simulink model "ES101A_DiagcMgr"  (R2013b)
settings: Solver=ode45  StartTime=0.0  StopTime=0.44  RelTol=1e-3
values from neighbouring files (symbols this model uses):
  BrdgVltg = DataDict.IpSignal    [ES101A_DiagcMgr_DataDict.m]
  DEM_CLEAR_PENDING = DataDict.Constant    [ES101A_DiagcMgr_DataDict.m]
  DEM_DTC_GROUP_ALL_DTCS = DataDict.Constant    [ES101A_DiagcMgr_DataDict.m]
  DFTAGICNTR_CNT_U08 = DataDict.Constant    [ES101A_DiagcMgr_DataDict.m]
  DIAGCMGR_NTCINFOSTSTESTFAILD_CNT_U08 = DataDict.Constant    [ES101A_DiagcMgr_DataDict.m]
  DIAGCMGR_NTCINFOSTSTESTFAILDTHISIGNCYC_CNT_U08 = DataDict.Constant    [ES101A_DiagcMgr_DataDict.m]
  DIAGCMGR_NTCINFOSTSTESTNOTCMPLTHISIGNCYC_CNT_U08 = DataDict.Constant    [ES101A_DiagcMgr_DataDict.m]
  DiagcMgrFltResp = DataDict.Calibration    [ES101A_DiagcMgr_DataDict.m]
  DiagcMgrNtcFltAry = DataDict.NVM    [ES101A_DiagcMgr_DataDict.m]
  DIAGCSTSCTRLDSHTDWNFLTPRSNT_CNT_U16 = DataDict.Constant    [ES101A_DiagcMgr_DataDict.m]
  DIAGCSTSDFTHWAG_CNT_U16 = DataDict.Constant    [ES101A_DiagcMgr_DataDict.m]
  DIAGCSTSDFTHWAGSERLCOMEXPRTVAL_CNT_U16 = DataDict.Constant    [ES101A_DiagcMgr_DataDict.m]
  DIAGCSTSDFTVEHSPD_CNT_U16 = DataDict.Constant    [ES101A_DiagcMgr_DataDict.m]
  DIAGCSTSININVAL_CNT_U16 = DataDict.Constant    [ES101A_DiagcMgr_DataDict.m]
  DIAGCSTSIVTR1INACTV_CNT_U16 = DataDict.Constant    [ES101A_DiagcMgr_DataDict.m]
  DIAGCSTSIVTR2INACTV_CNT_U16 = DataDict.Constant    [ES101A_DiagcMgr_DataDict.m]
  DIAGCSTSLIMDTPRFMNC_CNT_U16 = DataDict.Constant    [ES101A_DiagcMgr_DataDict.m]
  DIAGCSTSRAMPTOZEROFLTPRSNT_CNT_U16 = DataDict.Constant    [ES101A_DiagcMgr_DataDict.m]
  DIAGCSTSWHLIMBREJCTNDI_CNT_U16 = DataDict.Constant    [ES101A_DiagcMgr_DataDict.m]
  DTCIDXSTSFAIL_CNT_U08 = DataDict.Constant    [ES101A_DiagcMgr_DataDict.m]
  DTCIDXSTSNONTC_CNT_U08 = DataDict.Constant    [ES101A_DiagcMgr_DataDict.m]
  DTCIDXSTSNORES_CNT_U08 = DataDict.Constant    [ES101A_DiagcMgr_DataDict.m]
  DTCIDXSTSPASS_CNT_U08 = DataDict.Constant    [ES101A_DiagcMgr_DataDict.m]
  DTCIDXSTSUPDCFMD_CNT_U08 = DataDict.Constant    [ES101A_DiagcMgr_DataDict.m]
  ELECGLBPRM_IVTRCNT_CNT_U08 = DataDict.ConfigParam    [ES101A_DiagcMgr_DataDict.m]
  FLTINJ_DIAGCMGR_DIAGCSTSIVTR1INACTV = DataDict.Constant    [ES101A_DiagcMgr_DataDict.m]
  FLTINJ_DIAGCMGR_DIAGCSTSIVTR2INACTV = DataDict.Constant    [ES101A_DiagcMgr_DataDict.m]
  HwTq = DataDict.IpSignal    [ES101A_DiagcMgr_DataDict.m]
  IgnCntr = DataDict.IpSignal    [ES101A_DiagcMgr_DataDict.m]
  MAXDEBCNTRVAL_CNT_S16 = DataDict.Constant    [ES101A_DiagcMgr_DataDict.m]
  MAXRAMPRATE_ULSPERSEC_F32 = DataDict.Constant    [ES101A_DiagcMgr_DataDict.m]
  MINDEBCNTRVAL_CNT_S16 = DataDict.Constant    [ES101A_DiagcMgr_DataDict.m]
  MINRAMPRATE_ULSPERSEC_F32 = DataDict.Constant    [ES101A_DiagcMgr_DataDict.m]
  SCAMOTTQCMDTOONE_ULS_F32 = DataDict.Constant    [ES101A_DiagcMgr_DataDict.m]
  SCAMOTTQCMDTOZERO_ULS_F32 = DataDict.Constant    [ES101A_DiagcMgr_DataDict.m]
  SysSt = DataDict.IpSignal    [ES101A_DiagcMgr_DataDict.m]
  VehSpd = DataDict.IpSignal    [ES101A_DiagcMgr_DataDict.m]
undefined symbols (not defined in the file or in its folder): ActvMotTqCmdSca, ActvRampRate, AgiCntr, Dem_DTCFormatType, Dem_DTCOriginType, Dem_EventStatusType, DiagcData, DiagcMgrNtcMap, DiagcSts, DtcEnaMask, EcuT, HistNtcFltAry, MicroDiagcData, MotTq, NtcNr, NtcNrWithResd1, NtcStInfo, ProxySetNtcData, Sts, SysSt1, TOTNROFDTC_CNT_U08
libraries: simulink x151, FloatToFixd x5, NxtrNvM x4
(part 2 of 13)

== system ES101A_DiagcMgr/DiagcMgr/ClrSnpshtData ==
  Function : TriggerPort  TriggerType=function-call  OutputDataType=double
  Constant : Constant  OutDataTypeStr=uint8
  CopyRight2 : Subsystem  Description=|  mask(Copyright Information){none=on}
      | Copyright info block.                                               
      |                                                                     
      | Place copyright information at the top of every subsystem in design.
      mask prompts: none "No parameters"
      mask help: Place copyright information at the top of every subsystem in design.
      mask Display:
      | NxtrConf = 'Nexteer Confidential';
      | 
      | sys = bdroot; %handle for the current model ("system")
      | first = get_param(sys,'Created');
      | first = first(end-3:end);  %year is last four digits
      | 
      | last = get_param(sys,'LastModifiedDate');
      | if isempty(last)
      |     last = datestr(now,'yyyy');
      | else
      |     last = last(end-3:end);
      | end
      | 
      | if strcmp(first,last)
      |     fprintf('%s -- Copyright %s Nexteer',NxtrConf,first)
      | else
      |     fprintf('%s -- %s%s- %s Nexteer',NxtrConf,char(169),first,last)
      | end
  Data Store Read1 : DataStoreRead  DataStoreName=SnpshtDataAry
  Set Ram Block Status : NxtrNvM/Set Ram Block Status  FuncName=Set Ram Block Status  NvMBlockName=SnpShtDataAry  VoidFuncRtn=on  BlockChanged_DSN=NvMSRBS_BlockChanged  Return_DSN=NvMSRBS_Return
      settings: AttributesFormatString=%<FuncName>
  Subsystem : Subsystem
  Width : Width  DataType=uint8
  wires:
  Width/1 -> Subsystem/1(Length of Snapshot Array)
  Data Store Read1/1 -> Width/1
  Constant/1 -> Set Ram Block Status/1

== system ES101A_DiagcMgr/DiagcMgr/CopyRight2 ==

== system ES101A_DiagcMgr/DiagcMgr/DiagcMgrIninCore ==
  note: ProxySetNtcData and DiagcData
      | are not inputs, outputs or arguments to the
      | DiagcMgrIninCore. They are being used for
      | modelling purpose to show that the data is
      | being written to the respective structs.
  AppIdx_ArgIn : Inport
  NtcInfoArySize : Inport  Port=2
  NtcInfoAry_ArgIn : Inport  Port=3
  DiagcData : Inport  Port=4
  ProxySetNtcData : Inport  Port=5
  Function : TriggerPort  TriggerType=function-call  OutputDataType=double
  CopyRight2 : Subsystem  Description=|  mask(Copyright Information){none=on}
      | Copyright info block.                                               
      |                                                                     
      | Place copyright information at the top of every subsystem in design.
      mask prompts: none "No parameters"
      mask help: Place copyright information at the top of every subsystem in design.
      mask Display:
      | NxtrConf = 'Nexteer Confidential';
      | 
      | sys = bdroot; %handle for the current model ("system")
      | first = get_param(sys,'Created');
      | first = first(end-3:end);  %year is last four digits
      | 
      | last = get_param(sys,'LastModifiedDate');
      | if isempty(last)
      |     last = datestr(now,'yyyy');
      | else
      |     last = last(end-3:end);
      | end
      | 
      | if strcmp(first,last)
      |     fprintf('%s -- Copyright %s Nexteer',NxtrConf,first)
      | else
      |     fprintf('%s -- %s%s- %s Nexteer',NxtrConf,char(169),first,last)
      | end
  Initialize the NtcInfo Array : Subsystem  Priority=2
      settings: AttributesFormatString=Priority = %<Priority>
  Update DiagcSts and DiagcMgrActv : Subsystem  RequirementInfo="{'linktype_rmi_doors' '0000c474 (/ESG Group/FDD Module Requirements/EA4 Specific/ES101A_DiagcMgr)' '#ES101A_288' 'true' 'REQ:  ES101A_288' '' ; 'linktype_rmi_doors' '0000c474 (/ESG Group/FDD Module Requirements/EA4 Specific/ES101A_DiagcMgr)' '#ES101A_147' 'true' 'REQ:  ES101A_147' '' } %GIDa_8493db0a_cdf8_4c0c_9032_5c31bd2188ab"  Priority=3
      settings: AttributesFormatString=Priority = %<Priority>
  Update NtcInfoAry From NvM : Subsystem  Priority=1
      settings: AttributesFormatString=Priority = %<Priority>
  ProxySetNtcData_ArgOut : Outport
  DiagcData_ArgOut : Outport  Port=2
  NtcInfoAry_ArgOut : Outport  Port=3
  wires:
  Update DiagcSts and DiagcMgrActv/1(ProxySetNtcData_ArgOut) -> ProxySetNtcData_ArgOut/1
  Update DiagcSts and DiagcMgrActv/2(DiagcData_ArgOut) -> DiagcData_ArgOut/1
  NtcInfoArySize/1 -> Initialize the NtcInfo Array/1(NtcInfoArySize)
  Initialize the NtcInfo Array/1(NtcInfoAry_ArgOut) -> NtcInfoAry_ArgOut/1
  AppIdx_ArgIn/1 -> Update NtcInfoAry From NvM/1(AppIdx_ArgIn)
  NtcInfoAry_ArgIn/1 -> Update NtcInfoAry From NvM/2(NtcInfoAry_ArgIn)
  ProxySetNtcData/1 -> Update DiagcSts and DiagcMgrActv/1(ProxySetNtcData)
  DiagcData/1 -> Update DiagcSts and DiagcMgrActv/2(DiagcData)
  Update NtcInfoAry From NvM/1(NtcInfoAry_ArgOut) -> [NtcInfoAry]
  [NtcInfoAry] -> Initialize the NtcInfo Array/2(NtcInfoAry_ArgIn)

== system ES101A_DiagcMgr/DiagcMgr/DiagcMgrPer1 ==
  note: SysDiRampRate and SysDiMotTqCmdSca have their initial output set as
      | 0.1 UlsPerSec and 1 respectively.
  note: Design Consideration:
      |
      | ES101A_v2.X.0 assumes that no loop faster than 2ms can set faults.
      |
      | OutpDiagcSts, OutpActvRampRate and OutpActvMotTqCmdSca are initialized to
      | the default values.
      |
      | Default values of OutpDiagcSts is DIAGCSTSIVTR2INACTV_CNT_U16 if the program is a single inverter configuration.
      | else DIAGCSTSININVAL_CNT_U16 if the program is a dual inverter configuration.
      |
      | Default values of OutpRampRate is MINRAMPRATE_ULSPERSEC_F32.
      |
      | Default values of OutpMotTqCmdSca is SCAMOTTQCMDTOONE_ULS_F32.
      |
      | Need to call the server runnable GetDiagcDataApplX to get the DiagcMgrDiagcSts,
      | DiagcMgrActvRampRate and DiagcMgrActvMotTqCmdSca
      |
      | DiagcMgrPer1 udpates the OutpDiagcSts with the
      | ORed values of ALL application's DiagcMgrDiagcStsX
      |
      | DiagcMgrPer1 udpates the OutpActvRampRate with the
      | MAX value of ALL application's DiagcMgrRampRateX.
      |
      | DiagcMgrPer1 udpates the OutpActvMotTqCmdSca with the
      | MIN value of ALL application's DiagcMgrMotTqCmdScaX
  Function : TriggerPort  TriggerType=function-call
  CopyRight2 : Subsystem  Description=|  mask(Copyright Information){none=on}
      | Copyright info block.                                               
      |                                                                     
      | Place copyright information at the top of every subsystem in design.
      mask prompts: none "No parameters"
      mask help: Place copyright information at the top of every subsystem in design.
      mask Display:
      | NxtrConf = 'Nexteer Confidential';
      | 
      | sys = bdroot; %handle for the current model ("system")
      | first = get_param(sys,'Created');
      | first = first(end-3:end);  %year is last four digits
      | 
      | last = get_param(sys,'LastModifiedDate');
      | if isempty(last)
      |     last = datestr(now,'yyyy');
      | else
      |     last = last(end-3:end);
      | end
      | 
      | if strcmp(first,last)
      |     fprintf('%s -- Copyright %s Nexteer',NxtrConf,first)
      | else
      |     fprintf('%s -- %s%s- %s Nexteer',NxtrConf,char(169),first,last)
      | end
  Update OutpDiagcData : Subsystem  RequirementInfo={} %GIDa_85c462ac_a7f2_40f7_9507_c2fa4f4de765  Priority=2  TreatAsAtomicUnit=on
      settings: AttributesFormatString=|
      | Priority = %<Priority>
      | %<Description>
  Update the Reduced Performance Outputs : Subsystem  Priority=2
      settings: AttributesFormatString=Priority = %<Priority>
  SysDiRampRate : Outport  InitialOutput=0.1
  SysDiMotTqCmdSca : Outport  Port=2  OutMin=[0]  OutMax=[1]  InitialOutput=1
  SysStFltOutpReqDi : Outport  Port=3
  DiagcStsLimdTPrfmnc : Outport  Port=4
  DiagcStsIvtr1Inactv : Outport  Port=5
  DiagcStsIvtr2Inactv : Outport  Port=6
  DiagcStsDftHwAg : Outport  RequirementInfo={} %GIDa_cebdabc8_1fab_4827_8ce2_641fe406cf61  Port=7
  DiagcStsDftVehSpd : Outport  RequirementInfo={} %GIDa_5ce1feaf_f885_43d9_a11b_961b529a5fef  Port=8
  DiagcStsDftHwAgSerlComExprtVal : Outport  RequirementInfo={} %GIDa_e0e4e2a8_addf_43dd_a724_2e2318a08aac  Port=9
  DiagcStsWhlImbRejctnDi : Outport  RequirementInfo={} %GIDa_d2eab3b7_33f5_4627_ba04_dc7cade08e2d  Port=10
  DiagcStsCtrldShtDwnFltPrsnt : Outport  RequirementInfo={} %GIDa_78682114_6521_49d0_bf72_17a6b6e216ee  Port=11
  wires:
  Update the Reduced Performance Outputs/1(SysDiRampRate) -> SysDiRampRate/1
  Update the Reduced Performance Outputs/2(SysDiMotTqCmdSca) -> SysDiMotTqCmdSca/1
  Update the Reduced Performance Outputs/3(SysStFltOutpReqDi) -> SysStFltOutpReqDi/1
  Update the Reduced Performance Outputs/4(DiagcStsLimdTPrfmnc) -> DiagcStsLimdTPrfmnc/1
  Update the Reduced Performance Outputs/5(DiagcStsIvtr1Inactv) -> DiagcStsIvtr1Inactv/1
  Update the Reduced Performance Outputs/6(DiagcStsIvtr2Inactv) -> DiagcStsIvtr2Inactv/1
  Update the Reduced Performance Outputs/7(DiagcStsDftHwAg) -> DiagcStsDftHwAg/1
  Update the Reduced Performance Outputs/8(DiagcStsDftVehSpd) -> DiagcStsDftVehSpd/1
  Update the Reduced Performance Outputs/9(DiagcStsDftHwAgSerlComExprtVal) -> DiagcStsDftHwAgSerlComExprtVal/1
  Update the Reduced Performance Outputs/10(DiagcStsWhlImbRejctnDi) -> DiagcStsWhlImbRejctnDi/1
  Update the Reduced Performance Outputs/11(DiagcStsCtrldShtDwnFltPrsnt) -> DiagcStsCtrldShtDwnFltPrsnt/1
  Update OutpDiagcData/1(OutpDiagcSts) -> [OutpDiagcSts]
  Update OutpDiagcData/3(OutpMotTqCmdSca) -> [OutpMotTqCmdSca]
  Update OutpDiagcData/2(OutpRampRate) -> [OutpRampRate]
  [OutpRampRate] -> Update the Reduced Performance Outputs/2(OutpRampRate)
  [OutpMotTqCmdSca] -> Update the Reduced Performance Outputs/3(OutpMotTqCmdSca)
  [OutpDiagcSts] -> Update the Reduced Performance Outputs/1(OutpDiagcSts)

== system ES101A_DiagcMgr/DiagcMgr/DiagcMgrPer2 ==
  note: Limitation of the design:
      | Suppose, as an example, we have NTCs 5,6,7 and 8 mapped to a DTC 4:
      | If NTCs 5,6,7 have a status of NoRes and 8 Reaches a status of Failed, the DTC is
      | updated to show a status of Failed.
      | If the NTC 8 is a recoverable NTC, then happens to reach a state of Passed,
      | the DtcIdxSts will show a status of NoRes and the DEM will still show that the DTC has Failed.
  Function : TriggerPort  TriggerType=function-call
  Clear All DTCs : Subsystem  RequirementInfo="{'linktype_rmi_doors' '0000c474 (/ESG Group/FDD Module Requirements/EA4 Specific/ES101A_DiagcMgr)' '#ES101A_318' 'true' 'REQ:  ES101A_318' '' } %GIDa_daa6a456_375f_4596_a22c_ed37d4d53311"
  CopyRight2 : Subsystem  Description=|  mask(Copyright Information){none=on}
      | Copyright info block.                                               
      |                                                                     
      | Place copyright information at the top of every subsystem in design.
      mask prompts: none "No parameters"
      mask help: Place copyright information at the top of every subsystem in design.
      mask Display:
      | NxtrConf = 'Nexteer Confidential';
      | 
      | sys = bdroot; %handle for the current model ("system")
      | first = get_param(sys,'Created');
      | first = first(end-3:end);  %year is last four digits
      | 
      | last = get_param(sys,'LastModifiedDate');
      | if isempty(last)
      |     last = datestr(now,'yyyy');
      | else
      |     last = last(end-3:end);
      | end
      | 
      | if strcmp(first,last)
      |     fprintf('%s -- Copyright %s Nexteer',NxtrConf,first)
      | else
      |     fprintf('%s -- %s%s- %s Nexteer',NxtrConf,char(169),first,last)
      | end
  Data Store Read : DataStoreRead  DataStoreName=PrevClrDtcFlg
  Data Store Read1 : DataStoreRead  DataStoreName=ClrDiagcFlg
  If : If  NumInputs=2  IfExpression=u1 ~= u2
  Normal Periodic Processing : Subsystem  RequirementInfo="{'linktype_rmi_doors' '0000c474 (/ESG Group/FDD Module Requirements/EA4 Specific/ES101A_DiagcMgr)' '#ES101A_322' 'true' 'REQ:  ES101A_322' '' ; 'linktype_rmi_doors' '0000c474 (/ESG Group/FDD Module Requirements/EA4 Specific/ES101A_DiagcMgr)' '#ES101A_308' 'true' 'REQ:  ES101A_308' '' } %GIDa_fa1cf601_71d2_4de3_81ca_c465534cf8bb"
  wires:
  Data Store Read1/1 -> If/1
  Data Store Read/1 -> If/2
  If/1 -> Clear All DTCs/Action
  If/2 -> Normal Periodic Processing/Action

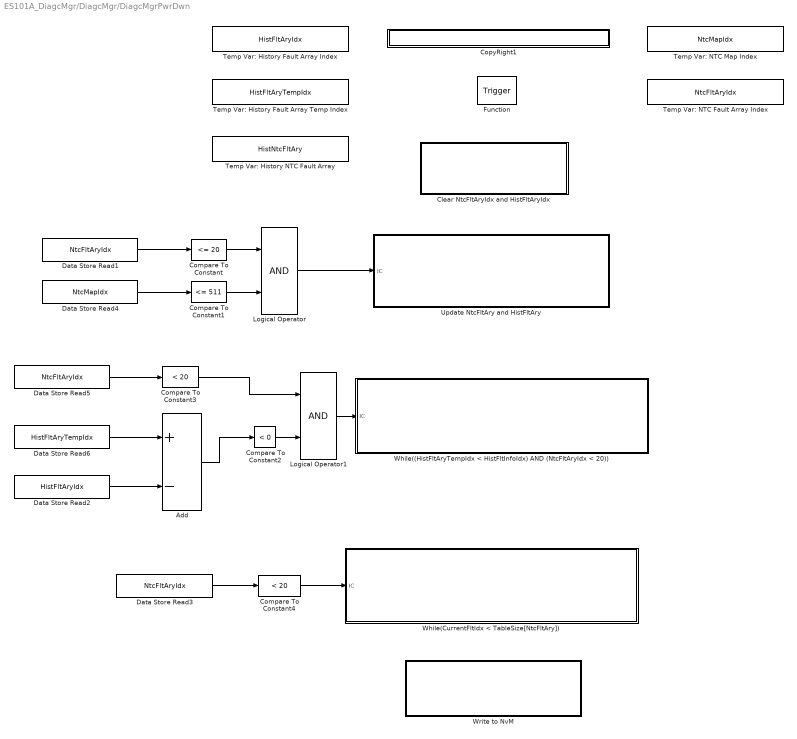
== system ES101A_DiagcMgr/DiagcMgr/DiagcMgrPwrDwn ==
  Function : TriggerPort  TriggerType=function-call
  Add : Sum  Inputs=+-
  Clear NtcFltAryIdx and HistFltAryIdx : Subsystem  Priority=1
      settings: AttributesFormatString=Priority = %<Priority>
  Compare To Constant : simulink/Logic and Bit Operations/Compare To Constant  relop=<=  const=20  OutDataTypeStr=boolean
  Compare To Constant1 : simulink/Logic and Bit Operations/Compare To Constant  relop=<=  const=511  OutDataTypeStr=boolean
  Compare To Constant2 : simulink/Logic and Bit Operations/Compare To Constant  relop=<  const=0  OutDataTypeStr=boolean
  Compare To Constant3 : simulink/Logic and Bit Operations/Compare To Constant  relop=<  const=20  OutDataTypeStr=boolean
  Compare To Constant4 : simulink/Logic and Bit Operations/Compare To Constant  relop=<  const=20  OutDataTypeStr=boolean
  CopyRight1 : Subsystem  Description=|  mask(Copyright Information){none=on}
      | Copyright info block.                                               
      |                                                                     
      | Place copyright information at the top of every subsystem in design.
      mask prompts: none "No parameters"
      mask help: Place copyright information at the top of every subsystem in design.
      mask Display:
      | NxtrConf = 'Nexteer Confidential';
      | 
      | sys = bdroot; %handle for the current model ("system")
      | first = get_param(sys,'Created');
      | first = first(end-3:end);  %year is last four digits
      | 
      | last = get_param(sys,'LastModifiedDate');
      | if isempty(last)
      |     last = datestr(now,'yyyy');
      | else
      |     last = last(end-3:end);
      | end
      | 
      | if strcmp(first,last)
      |     fprintf('%s -- Copyright %s Nexteer',NxtrConf,first)
      | else
      |     fprintf('%s -- %s%s- %s Nexteer',NxtrConf,char(169),first,last)
      | end
  Data Store Read1 : DataStoreRead  DataStoreName=NtcFltAryIdx
  Data Store Read2 : DataStoreRead  DataStoreName=HistFltAryIdx
  Data Store Read3 : DataStoreRead  DataStoreName=NtcFltAryIdx
  Data Store Read4 : DataStoreRead  DataStoreName=NtcMapIdx
  Data Store Read5 : DataStoreRead  DataStoreName=NtcFltAryIdx
  Data Store Read6 : DataStoreRead  DataStoreName=HistFltAryTempIdx
  Logical Operator : Logic  AllPortsSameDT=off  OutDataTypeStr=boolean
  Logical Operator1 : Logic  AllPortsSameDT=off  OutDataTypeStr=boolean
  Temp Var: History Fault Array Index : DataStoreMemory  DataStoreName=HistFltAryIdx  ReadBeforeWriteMsg=warning  WriteAfterWriteMsg=warning  WriteAfterReadMsg=warning  InitialValue=19  OutDataTypeStr=uint8
  Temp Var: History Fault Array Temp Index : DataStoreMemory  DataStoreName=HistFltAryTempIdx  ReadBeforeWriteMsg=warning  WriteAfterWriteMsg=warning  WriteAfterReadMsg=warning  InitialValue=1  OutDataTypeStr=uint8
  Temp Var: History NTC Fault Array : DataStoreMemory  RequirementInfo={} %GIDa_eaafd789_c2c3_4d7f_bafd_485e89611a26  DataStoreName=HistNtcFltAry  InitialValue=[0 0 0 0 0 0 0 0 0 0 0 0 0 0 0 0 0 0 0 0]  OutDataTypeStr=Bus: NtcFltInfoRec1  Dimensions=20
  Temp Var: NTC Fault Array Index : DataStoreMemory  DataStoreName=NtcFltAryIdx  ReadBeforeWriteMsg=warning  WriteAfterWriteMsg=warning  WriteAfterReadMsg=warning  InitialValue=19  OutDataTypeStr=uint8
  Temp Var: NTC Map Index : DataStoreMemory  DataStoreName=NtcMapIdx  ReadBeforeWriteMsg=warning  WriteAfterWriteMsg=warning  WriteAfterReadMsg=warning  InitialValue=1  OutDataTypeStr=uint8
  Update NtcFltAry and HistFltAry : Subsystem  Priority=2
      settings: AttributesFormatString=Priority = %<Priority>
  While((HistFltAryTempIdx < HistFltInfoIdx) AND (NtcFltAryIdx < 20)) : Subsystem  Priority=3  TreatAsAtomicUnit=on
      settings: AttributesFormatString=Priority = %<Priority>
  While(CurrentFltIdx < TableSize[NtcFltAry]) : Subsystem  Priority=4  TreatAsAtomicUnit=on
      settings: AttributesFormatString=Priority = %<Priority>
  Write to NvM : Subsystem  Priority=5
      settings: AttributesFormatString=Priority = %<Priority>
  wires:
  Data Store Read3/1 -> Compare To Constant4/1
  Compare To Constant4/1 -> While(CurrentFltIdx < TableSize[NtcFltAry])/1(IC)
  Logical Operator/1 -> Update NtcFltAry and HistFltAry/1(IC)
  Data Store Read1/1 -> Compare To Constant/1
  Compare To Constant/1 -> Logical Operator/1
  Compare To Constant1/1 -> Logical Operator/2
  Data Store Read4/1 -> Compare To Constant1/1
  Data Store Read6/1 -> Add/1
  Data Store Read2/1 -> Add/2
  Add/1 -> Compare To Constant2/1
  Data Store Read5/1 -> Compare To Constant3/1
  Compare To Constant3/1 -> Logical Operator1/1
  Logical Operator1/1 -> While((HistFltAryTempIdx < HistFltInfoIdx) AND (NtcFltAryIdx < 20))/1(IC)
  Compare To Constant2/1 -> Logical Operator1/2

== system ES101A_DiagcMgr/DiagcMgr/GetNtcActvCore  ==
  note: SW Implementation:
      |
      | 	SW uses a switched case with ApplIdx as the input. The GetNtcInfoApplX is
      | 	called inside each of the switched case statements. Based on the application
      | 	index, the respective NtcInfoAryX is selected.
  note: Design Rationale:
      |
      | 	If an NTC that is not configured in the NTC Map is called by any application/component,
      | 	its application index would be read as 255 and it enters the default case in the above switch
      | 	statement. This would indicate that the NTC has a Not Active State.
  NtcNr_ArgIn : Inport
  Function : TriggerPort  TriggerType=function-call
  Bus Selector : BusSelector  OutputSignals=Sts
  Bus Selector3 : BusSelector  OutputSignals=ApplIdx,NtcInfoIdx
  Compare to Zero : simulink/Logic and Bit Operations/Compare To Zero  relop=~=  OutDataTypeStr=boolean
  Compare to Zero1 : simulink/Logic and Bit Operations/Compare To Zero  relop=~=  OutDataTypeStr=boolean
  CopyRight2 : Subsystem  Description=|  mask(Copyright Information){none=on}
      | Copyright info block.                                               
      |                                                                     
      | Place copyright information at the top of every subsystem in design.
      mask prompts: none "No parameters"
      mask help: Place copyright information at the top of every subsystem in design.
      mask Display:
      | NxtrConf = 'Nexteer Confidential';
      | 
      | sys = bdroot; %handle for the current model ("system")
      | first = get_param(sys,'Created');
      | first = first(end-3:end);  %year is last four digits
      | 
      | last = get_param(sys,'LastModifiedDate');
      | if isempty(last)
      |     last = datestr(now,'yyyy');
      | else
      |     last = last(end-3:end);
      | end
      | 
      | if strcmp(first,last)
      |     fprintf('%s -- Copyright %s Nexteer',NxtrConf,first)
      | else
      |     fprintf('%s -- %s%s- %s Nexteer',NxtrConf,char(169),first,last)
      | end
  DIAGCMGR_NTCINFOSTSTESTFAILDTHISIGNCYC_CNT_U08 : simulink/Logic and Bit Operations/Bitwise Operator  logicop=AND  UseBitMask=on  BitMask=DIAGCMGR_NTCINFOSTSTESTFAILDTHISIGNCYC_CNT_U08  BitMaskRealWorld=Stored Integer
  DIAGCMGR_NTCINFOSTSTESTFAILD_CNT_U08 : simulink/Logic and Bit Operations/Bitwise Operator  logicop=AND  UseBitMask=on  BitMask=DIAGCMGR_NTCINFOSTSTESTFAILD_CNT_U08  BitMaskRealWorld=Stored Integer
  Data Store Read2 : DataStoreRead  DataStoreName=DiagcMgrNtcMap  DataStoreElements=DiagcMgrNtcMap(:)
  Data Type Conversion : DataTypeConversion  OutDataTypeStr=uint16
  GetNtcInfoAppIX : Subsystem  TreatAsAtomicUnit=on
  Logical Operator : Logic  AllPortsSameDT=off  OutDataTypeStr=boolean
  Merge1 : Merge
  NTC Not Active : Subsystem  TreatAsAtomicUnit=on
  Selector1 : Selector  IndexMode=Zero-based  InputPortWidth=512  IndexOptions=Index vector (port)  Indices=[1 3]  OutputSizes=1
  Switch Case : SwitchCase  CaseConditions={X}
  NtcActv_ArgOut : Outport
  wires:
  DIAGCMGR_NTCINFOSTSTESTFAILD_CNT_U08/1 -> Compare to Zero/1
  DIAGCMGR_NTCINFOSTSTESTFAILDTHISIGNCYC_CNT_U08/1 -> Compare to Zero1/1
  Compare to Zero/1 -> Logical Operator/1
  Compare to Zero1/1 -> Logical Operator/2
  Logical Operator/1 -> NtcActv_ArgOut/1
  Data Store Read2/1 -> Selector1/1
  NtcNr_ArgIn/1 -> Data Type Conversion/1
  Data Type Conversion/1 -> Selector1/2
  Selector1/1 -> Bus Selector3/1
  Bus Selector3/1 -> Switch Case/1  "<ApplIdx>"
  Switch Case/1 -> GetNtcInfoAppIX/Action
  Bus Selector3/2 -> GetNtcInfoAppIX/1(NtcInfoIdx_ArgIn)  "<NtcInfoIdx>"
  Switch Case/2 -> NTC Not Active/Action
  GetNtcInfoAppIX/1(NtcInfo_ArgOut) -> Bus Selector/1
  NTC Not Active/1(Sts) -> Merge1/2
  Bus Selector/1 -> Merge1/1  "<Sts>"
  Merge1/1 -> DIAGCMGR_NTCINFOSTSTESTFAILDTHISIGNCYC_CNT_U08/1, DIAGCMGR_NTCINFOSTSTESTFAILD_CNT_U08/1

== system ES101A_DiagcMgr/DiagcMgr/GetNtcQlfrStsCore  ==
  note: Enumeration of SigQlfr1
      |         SIGQLFR_NORES   (0)
      |         SIGQLFR_PASSD    (1)
      |         SIGQLFR_FAILD      (2)
  note: SW Implementation:
      |
      | 	SW uses a switched case with ApplIdx as the input. The GetNtcInfoApplX is
      | 	called inside each of the switched case statements. Based on the application
      | 	index, the respective NtcInfoAryX is selected.
  note: Design Rationale:
      |
      | 	If an NTC that is not configured in the NTC Map is called by any application/component,
      | 	its application index would be read as 255 and it enters the default case in the above switch
      | 	statement. This would indicate that the NTC has a No Result State.
  NtcNr_ArgIn : Inport
  Function : TriggerPort  TriggerType=function-call
  Bus Selector : BusSelector  OutputSignals=Sts
  Bus Selector3 : BusSelector  OutputSignals=ApplIdx,NtcInfoIdx
  Compare to Zero : simulink/Logic and Bit Operations/Compare To Zero  relop=~=  OutDataTypeStr=boolean
  Compare to Zero1 : simulink/Logic and Bit Operations/Compare To Zero  relop=~=  OutDataTypeStr=boolean
  CopyRight2 : Subsystem  Description=|  mask(Copyright Information){none=on}
      | Copyright info block.                                               
      |                                                                     
      | Place copyright information at the top of every subsystem in design.
      mask prompts: none "No parameters"
      mask help: Place copyright information at the top of every subsystem in design.
      mask Display:
      | NxtrConf = 'Nexteer Confidential';
      | 
      | sys = bdroot; %handle for the current model ("system")
      | first = get_param(sys,'Created');
      | first = first(end-3:end);  %year is last four digits
      | 
      | last = get_param(sys,'LastModifiedDate');
      | if isempty(last)
      |     last = datestr(now,'yyyy');
      | else
      |     last = last(end-3:end);
      | end
      | 
      | if strcmp(first,last)
      |     fprintf('%s -- Copyright %s Nexteer',NxtrConf,first)
      | else
      |     fprintf('%s -- %s%s- %s Nexteer',NxtrConf,char(169),first,last)
      | end
  DIAGCMGR_NTCINFOSTSTESTFAILD_CNT_U08 : simulink/Logic and Bit Operations/Bitwise Operator  logicop=AND  UseBitMask=on  BitMask=DIAGCMGR_NTCINFOSTSTESTFAILD_CNT_U08  BitMaskRealWorld=Stored Integer
  DIAGCMGR_NTCINFOSTSTESTNOTCMPLTHISIGNCYC_CNT_U08 : simulink/Logic and Bit Operations/Bitwise Operator  logicop=AND  UseBitMask=on  BitMask=DIAGCMGR_NTCINFOSTSTESTNOTCMPLTHISIGNCYC_CNT_U08  BitMaskRealWorld=Stored Integer
  Data Store Read2 : DataStoreRead  DataStoreName=DiagcMgrNtcMap  DataStoreElements=DiagcMgrNtcMap(:)
  Data Type Conversion : DataTypeConversion  OutDataTypeStr=uint16
  GetNtcInfoAppIX : Subsystem  TreatAsAtomicUnit=on
  If : If  NumInputs=2  IfExpression=u1 == 1  ElseIfExpressions=u2 == 0
  Merge : Merge  Inputs=3
  Merge1 : Merge
  No Result State : Subsystem  TreatAsAtomicUnit=on
  SIGQLFR_FAILD : Subsystem  TreatAsAtomicUnit=on
  SIGQLFR_NORES : Subsystem  TreatAsAtomicUnit=on
  SIGQLFR_PASSD : Subsystem  TreatAsAtomicUnit=on
  Selector1 : Selector  IndexMode=Zero-based  InputPortWidth=512  IndexOptions=Index vector (port)  Indices=[1 3]  OutputSizes=1
  Switch Case : SwitchCase  CaseConditions={X}
  NtcQlfr_ArgOut : Outport
  wires:
  DIAGCMGR_NTCINFOSTSTESTNOTCMPLTHISIGNCYC_CNT_U08/1 -> Compare to Zero/1
  DIAGCMGR_NTCINFOSTSTESTFAILD_CNT_U08/1 -> Compare to Zero1/1
  Merge/1 -> NtcQlfr_ArgOut/1
  SIGQLFR_NORES/1(NtcQlfr) -> Merge/1
  SIGQLFR_PASSD/1(NtcQlfr) -> Merge/2
  SIGQLFR_FAILD/1(NtcQlfr) -> Merge/3
  If/3 -> SIGQLFR_FAILD/Action
  If/2 -> SIGQLFR_PASSD/Action
  If/1 -> SIGQLFR_NORES/Action
  Compare to Zero/1 -> If/1
  Compare to Zero1/1 -> If/2
  Data Store Read2/1 -> Selector1/1
  NtcNr_ArgIn/1 -> Data Type Conversion/1
  Data Type Conversion/1 -> Selector1/2
  Selector1/1 -> Bus Selector3/1
  Bus Selector3/1 -> Switch Case/1  "<ApplIdx>"
  Switch Case/1 -> GetNtcInfoAppIX/Action
  Bus Selector3/2 -> GetNtcInfoAppIX/1(NtcInfoIdx_ArgIn)  "<NtcInfoIdx>"
  Switch Case/2 -> No Result State/Action
  GetNtcInfoAppIX/1(NtcInfo_ArgOut) -> Bus Selector/1
  No Result State/1(Sts) -> Merge1/2
  Bus Selector/1 -> Merge1/1  "<Sts>"
  Merge1/1 -> DIAGCMGR_NTCINFOSTSTESTFAILD_CNT_U08/1, DIAGCMGR_NTCINFOSTSTESTNOTCMPLTHISIGNCYC_CNT_U08/1

== system ES101A_DiagcMgr/DiagcMgr/GetNtcStsCore ==
  note: SW Implementation:
      |
      | 	SW uses a switched case with ApplIdx as the input. The GetNtcInfoApplX is
      | 	called inside each of the switched case statements. Based on the application
      | 	index, the respective NtcInfoAryX is selected.
  note: Design Rationale:
      |
      | 	If an NTC that is not configured in the NTC Map is called by any application/component,
      | 	its application index would be read as 255 and it enters the default case in the above switch
      | 	statement. This would indicate that the NTC Status has a Defult Value.
  NtcNr_ArgIn : Inport
  Function : TriggerPort  TriggerType=function-call
  Bus Selector : BusSelector  OutputSignals=Sts
  Bus Selector3 : BusSelector  OutputSignals=ApplIdx,NtcInfoIdx
  CopyRight2 : Subsystem  Description=|  mask(Copyright Information){none=on}
      | Copyright info block.                                               
      |                                                                     
      | Place copyright information at the top of every subsystem in design.
      mask prompts: none "No parameters"
      mask help: Place copyright information at the top of every subsystem in design.
      mask Display:
      | NxtrConf = 'Nexteer Confidential';
      | 
      | sys = bdroot; %handle for the current model ("system")
      | first = get_param(sys,'Created');
      | first = first(end-3:end);  %year is last four digits
      | 
      | last = get_param(sys,'LastModifiedDate');
      | if isempty(last)
      |     last = datestr(now,'yyyy');
      | else
      |     last = last(end-3:end);
      | end
      | 
      | if strcmp(first,last)
      |     fprintf('%s -- Copyright %s Nexteer',NxtrConf,first)
      | else
      |     fprintf('%s -- %s%s- %s Nexteer',NxtrConf,char(169),first,last)
      | end
  Data Store Read2 : DataStoreRead  DataStoreName=DiagcMgrNtcMap  DataStoreElements=DiagcMgrNtcMap(:)
  Data Type Conversion : DataTypeConversion  OutDataTypeStr=uint16
  GetNtcInfoAppIX : Subsystem  TreatAsAtomicUnit=on
  Merge1 : Merge
  NTC Default Status : Subsystem  TreatAsAtomicUnit=on
  Selector1 : Selector  IndexMode=Zero-based  InputPortWidth=512  IndexOptions=Index vector (port)  Indices=[1 3]  OutputSizes=1
  Switch Case : SwitchCase  CaseConditions={X}
  NtcInfoSts_ArgOut : Outport
  wires:
  Bus Selector/1 -> NtcInfoSts_ArgOut/1  "<Sts>"
  Data Store Read2/1 -> Selector1/1
  Selector1/1 -> Bus Selector3/1
  NtcNr_ArgIn/1 -> Data Type Conversion/1
  Data Type Conversion/1 -> Selector1/2
  Bus Selector3/1 -> Switch Case/1  "<ApplIdx>"
  Switch Case/1 -> GetNtcInfoAppIX/Action
  Bus Selector3/2 -> GetNtcInfoAppIX/1(NtcInfoIdx_ArgIn)  "<NtcInfoIdx>"
  Switch Case/2 -> NTC Default Status/Action
  NTC Default Status/1(Sts) -> Merge1/2
  GetNtcInfoAppIX/1(NtcInfo_ArgOut) -> Merge1/1
  Merge1/1 -> Bus Selector/1

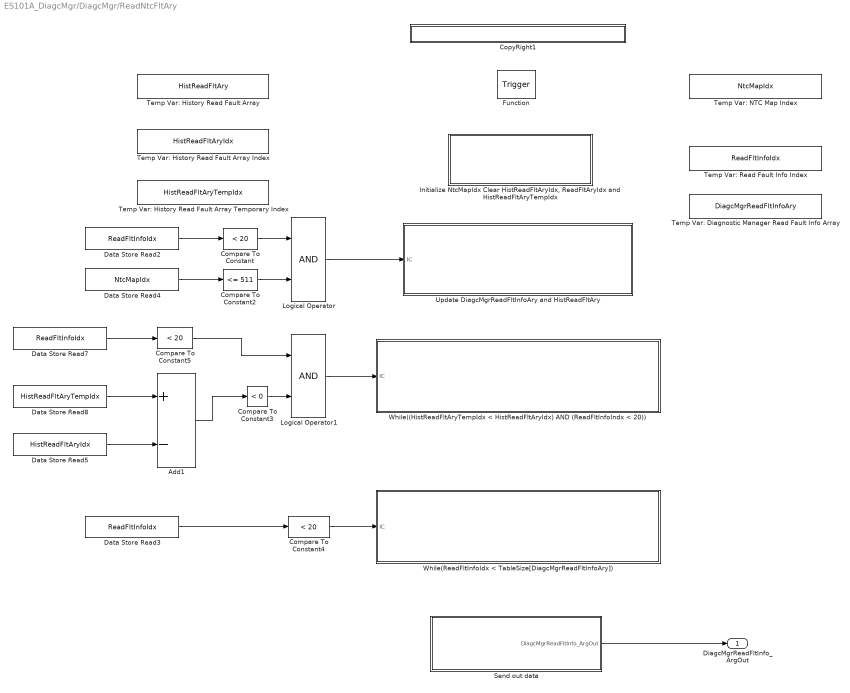
== system ES101A_DiagcMgr/DiagcMgr/ReadNtcFltAry ==
  Function : TriggerPort  TriggerType=function-call
  Add1 : Sum  Inputs=+-
  Compare To Constant : simulink/Logic and Bit Operations/Compare To Constant  relop=<  const=20  OutDataTypeStr=boolean
  Compare To Constant2 : simulink/Logic and Bit Operations/Compare To Constant  relop=<=  const=511  OutDataTypeStr=boolean
  Compare To Constant3 : simulink/Logic and Bit Operations/Compare To Constant  relop=<  const=0  OutDataTypeStr=boolean
  Compare To Constant4 : simulink/Logic and Bit Operations/Compare To Constant  relop=<  const=20  OutDataTypeStr=boolean
  Compare To Constant5 : simulink/Logic and Bit Operations/Compare To Constant  relop=<  const=20  OutDataTypeStr=boolean
  CopyRight1 : Subsystem  Description=|  mask(Copyright Information){none=on}
      | Copyright info block.                                               
      |                                                                     
      | Place copyright information at the top of every subsystem in design.
      mask prompts: none "No parameters"
      mask help: Place copyright information at the top of every subsystem in design.
      mask Display:
      | NxtrConf = 'Nexteer Confidential';
      | 
      | sys = bdroot; %handle for the current model ("system")
      | first = get_param(sys,'Created');
      | first = first(end-3:end);  %year is last four digits
      | 
      | last = get_param(sys,'LastModifiedDate');
      | if isempty(last)
      |     last = datestr(now,'yyyy');
      | else
      |     last = last(end-3:end);
      | end
      | 
      | if strcmp(first,last)
      |     fprintf('%s -- Copyright %s Nexteer',NxtrConf,first)
      | else
      |     fprintf('%s -- %s%s- %s Nexteer',NxtrConf,char(169),first,last)
      | end
  Data Store Read2 : DataStoreRead  DataStoreName=ReadFltInfoIdx
  Data Store Read3 : DataStoreRead  DataStoreName=ReadFltInfoIdx
  Data Store Read4 : DataStoreRead  DataStoreName=NtcMapIdx
  Data Store Read5 : DataStoreRead  DataStoreName=HistReadFltAryIdx
  Data Store Read7 : DataStoreRead  DataStoreName=ReadFltInfoIdx
  Data Store Read8 : DataStoreRead  DataStoreName=HistReadFltAryTempIdx
  "Initialize NtcMapIdx Clear HistReadFltAryIdx, ReadFltAryIdx and HistReadFltAryTempIdx" : Subsystem  Priority=1
      settings: AttributesFormatString=Priority = %<Priority>
  Logical Operator : Logic  AllPortsSameDT=off  OutDataTypeStr=boolean
  Logical Operator1 : Logic  AllPortsSameDT=off  OutDataTypeStr=boolean
  Send out data : Subsystem  Priority=6
      settings: AttributesFormatString=Priority = %<Priority>
  Temp Var: Diagnostic Manager Read Fault Info Array : DataStoreMemory  Description=|  RequirementInfo={} %GIDa_08928bd1_0b5a_40ca_b070_77c54a43db14  DataStoreName=DiagcMgrReadFltInfoAry  InitialValue=[0 0 0 0 0 0 0 0 0 0 0 0 0 0 0 0 0 0 0 0]  OutDataTypeStr=Bus: NtcFltInfoRec1  Dimensions=20
      | For Simulation Only. The output DiagcMgrReadFltInfoAry_ArgOut is
      | an array of structure that can only be defined using a DataStore block
      | in the model.
      settings: AttributesFormatString=%<Description>
  Temp Var: History Read Fault Array : DataStoreMemory  RequirementInfo={} %GIDa_4423747c_d3fb_471c_bd19_aa7473b94f03  DataStoreName=HistReadFltAry  InitialValue=[0 0 0 0 0 0 0 0 0 0 0 0 0 0 0 0 0 0 0 0]  OutDataTypeStr=Bus: NtcFltInfoRec1  Dimensions=20
  Temp Var: History Read Fault Array Index : DataStoreMemory  DataStoreName=HistReadFltAryIdx  ReadBeforeWriteMsg=warning  WriteAfterWriteMsg=warning  WriteAfterReadMsg=warning  InitialValue=1  OutDataTypeStr=uint8
  Temp Var: History Read Fault Array Temporary Index : DataStoreMemory  DataStoreName=HistReadFltAryTempIdx  ReadBeforeWriteMsg=warning  WriteAfterWriteMsg=warning  WriteAfterReadMsg=warning  InitialValue=1  OutDataTypeStr=uint8
  "Temp Var: NTC Map Index " : DataStoreMemory  DataStoreName=NtcMapIdx  ReadBeforeWriteMsg=warning  WriteAfterWriteMsg=warning  WriteAfterReadMsg=warning  InitialValue=1  OutDataTypeStr=uint8
  Temp Var: Read Fault Info Index : DataStoreMemory  DataStoreName=ReadFltInfoIdx  ReadBeforeWriteMsg=warning  WriteAfterWriteMsg=warning  WriteAfterReadMsg=warning  InitialValue=1  OutDataTypeStr=uint8
  Update DiagcMgrReadFltInfoAry and HistReadFltAry : Subsystem  Priority=2
      settings: AttributesFormatString=Priority = %<Priority>
  While((HistReadFltAryTempIdx < HistReadFltAryIdx) AND (ReadFltInfoIndx < 20)) : Subsystem  Priority=3  TreatAsAtomicUnit=on
      settings: AttributesFormatString=Priority = %<Priority>
  While(ReadFltInfoIdx < TableSize[DiagcMgrReadFltInfoAry]) : Subsystem  Priority=5  TreatAsAtomicUnit=on
      settings: AttributesFormatString=Priority = %<Priority>
  DiagcMgrReadFltInfo_ArgOut : Outport
  wires:
  Send out data/1(DiagcMgrReadFltInfo_ArgOut) -> DiagcMgrReadFltInfo_ArgOut/1
  Data Store Read3/1 -> Compare To Constant4/1
  Compare To Constant4/1 -> While(ReadFltInfoIdx < TableSize[DiagcMgrReadFltInfoAry])/1(IC)
  Logical Operator1/1 -> While((HistReadFltAryTempIdx < HistReadFltAryIdx) AND (ReadFltInfoIndx < 20))/1(IC)
  Logical Operator/1 -> Update DiagcMgrReadFltInfoAry and HistReadFltAry/1(IC)
  Data Store Read2/1 -> Compare To Constant/1
  Compare To Constant/1 -> Logical Operator/1
  Compare To Constant2/1 -> Logical Operator/2
  Data Store Read4/1 -> Compare To Constant2/1
  Data Store Read8/1 -> Add1/1
  Data Store Read5/1 -> Add1/2
  Add1/1 -> Compare To Constant3/1
  Data Store Read7/1 -> Compare To Constant5/1
  Compare To Constant5/1 -> Logical Operator1/1
  Compare To Constant3/1 -> Logical Operator1/2

== system ES101A_DiagcMgr/DiagcMgr/ReadNtcInfoAndDebCntr ==
  note: SW Implementation:
      |
      | 	SW uses a switched case with ApplIdx as the input. The GetNtcInfoApplX is
      | 	called inside each of the switched case statements. Based on the application
      | 	index, the respective NtcInfoAryX is selected.
  NtcNr_ArgIn : Inport
  Function : TriggerPort  TriggerType=function-call
  ApplX : Subsystem  TreatAsAtomicUnit=on
  Bus Selector1 : BusSelector  OutputSignals=ApplIdx,NtcInfoIdx,DebCntrIdx
  CopyRight2 : Subsystem  Description=|  mask(Copyright Information){none=on}
      | Copyright info block.                                               
      |                                                                     
      | Place copyright information at the top of every subsystem in design.
      mask prompts: none "No parameters"
      mask help: Place copyright information at the top of every subsystem in design.
      mask Display:
      | NxtrConf = 'Nexteer Confidential';
      | 
      | sys = bdroot; %handle for the current model ("system")
      | first = get_param(sys,'Created');
      | first = first(end-3:end);  %year is last four digits
      | 
      | last = get_param(sys,'LastModifiedDate');
      | if isempty(last)
      |     last = datestr(now,'yyyy');
      | else
      |     last = last(end-3:end);
      | end
      | 
      | if strcmp(first,last)
      |     fprintf('%s -- Copyright %s Nexteer',NxtrConf,first)
      | else
      |     fprintf('%s -- %s%s- %s Nexteer',NxtrConf,char(169),first,last)
      | end
  Data Store Read2 : DataStoreRead  DataStoreName=DiagcMgrNtcMap  DataStoreElements=DiagcMgrNtcMap(:)
  Data Type Conversion : DataTypeConversion  OutDataTypeStr=uint16
  DoNothing : Subsystem  TreatAsAtomicUnit=on
  Selector1 : Selector  IndexMode=Zero-based  InputPortWidth=512  IndexOptions=Index vector (port)  Indices=[1 3]  OutputSizes=1
  Switch Case : SwitchCase  CaseConditions={X}
  NtcInfo_ArgOut : Outport
  DebCntr_ArgOut : Outport  Port=2
  wires:
  Switch Case/2 -> DoNothing/Action
  Bus Selector1/2 -> ApplX/1(NtcInfoIdx_ArgIn)  "<NtcInfoIdx>"
  Switch Case/1 -> ApplX/Action
  Bus Selector1/1 -> Switch Case/1  "<ApplIdx>"
  Data Type Conversion/1 -> Selector1/2
  NtcNr_ArgIn/1 -> Data Type Conversion/1
  Selector1/1 -> Bus Selector1/1
  ApplX/1(NtcInfo_ArgOut) -> NtcInfo_ArgOut/1
  Data Store Read2/1 -> Selector1/1
  Bus Selector1/3 -> ApplX/2(DebCntrIdx_ArgIn)  "<DebCntrIdx>"
  ApplX/2(DebCntr_ArgOut) -> DebCntr_ArgOut/1

== system ES101A_DiagcMgr/DiagcMgr/ReadSnpshtData ==
  Function : TriggerPort  TriggerType=function-call
  CopyRight1 : Subsystem  Description=|  mask(Copyright Information){none=on}
      | Copyright info block.                                               
      |                                                                     
      | Place copyright information at the top of every subsystem in design.
      mask prompts: none "No parameters"
      mask help: Place copyright information at the top of every subsystem in design.
      mask Display:
      | NxtrConf = 'Nexteer Confidential';
      | 
      | sys = bdroot; %handle for the current model ("system")
      | first = get_param(sys,'Created');
      | first = first(end-3:end);  %year is last four digits
      | 
      | last = get_param(sys,'LastModifiedDate');
      | if isempty(last)
      |     last = datestr(now,'yyyy');
      | else
      |     last = last(end-3:end);
      | end
      | 
      | if strcmp(first,last)
      |     fprintf('%s -- Copyright %s Nexteer',NxtrConf,first)
      | else
      |     fprintf('%s -- %s%s- %s Nexteer',NxtrConf,char(169),first,last)
      | end
  Send out data : Subsystem  Priority=1
      settings: AttributesFormatString=Priority = %<Priority>
  ReadSnpshtAry_ArgOut : Outport
  wires:
  Send out data/1(ReadSnpshtAry_ArgOut) -> ReadSnpshtAry_ArgOut/1

== system ES101A_DiagcMgr/DiagcMgr/RestoreNtcFltAryDft ==
  Function : TriggerPort  TriggerType=function-call  OutputDataType=double
  CopyRight2 : Subsystem  Description=|  mask(Copyright Information){none=on}
      | Copyright info block.                                               
      |                                                                     
      | Place copyright information at the top of every subsystem in design.
      mask prompts: none "No parameters"
      mask help: Place copyright information at the top of every subsystem in design.
      mask Display:
      | NxtrConf = 'Nexteer Confidential';
      | 
      | sys = bdroot; %handle for the current model ("system")
      | first = get_param(sys,'Created');
      | first = first(end-3:end);  %year is last four digits
      | 
      | last = get_param(sys,'LastModifiedDate');
      | if isempty(last)
      |     last = datestr(now,'yyyy');
      | else
      |     last = last(end-3:end);
      | end
      | 
      | if strcmp(first,last)
      |     fprintf('%s -- Copyright %s Nexteer',NxtrConf,first)
      | else
      |     fprintf('%s -- %s%s- %s Nexteer',NxtrConf,char(169),first,last)
      | end
  Data Store Read1 : DataStoreRead  DataStoreName=DiagcMgrNtcFltAry
  Subsystem : Subsystem
  Width : Width  DataType=uint8
  wires:
  Width/1 -> Subsystem/1(Length of NtcFltArray)
  Data Store Read1/1 -> Width/1

== system ES101A_DiagcMgr/DiagcMgr/RestoreSnpshtAryDft ==
  Function : TriggerPort  TriggerType=function-call  OutputDataType=double
  CopyRight2 : Subsystem  Description=|  mask(Copyright Information){none=on}
      | Copyright info block.                                               
      |                                                                     
      | Place copyright information at the top of every subsystem in design.
      mask prompts: none "No parameters"
      mask help: Place copyright information at the top of every subsystem in design.
      mask Display:
      | NxtrConf = 'Nexteer Confidential';
      | 
      | sys = bdroot; %handle for the current model ("system")
      | first = get_param(sys,'Created');
      | first = first(end-3:end);  %year is last four digits
      | 
      | last = get_param(sys,'LastModifiedDate');
      | if isempty(last)
      |     last = datestr(now,'yyyy');
      | else
      |     last = last(end-3:end);
      | end
      | 
      | if strcmp(first,last)
      |     fprintf('%s -- Copyright %s Nexteer',NxtrConf,first)
      | else
      |     fprintf('%s -- %s%s- %s Nexteer',NxtrConf,char(169),first,last)
      | end
  Data Store Read1 : DataStoreRead  DataStoreName=SnpshtDataAry
  Subsystem : Subsystem
  Width : Width  DataType=uint8
  wires:
  Data Store Read1/1 -> Width/1
  Width/1 -> Subsystem/1(Length of Snapshot Array)

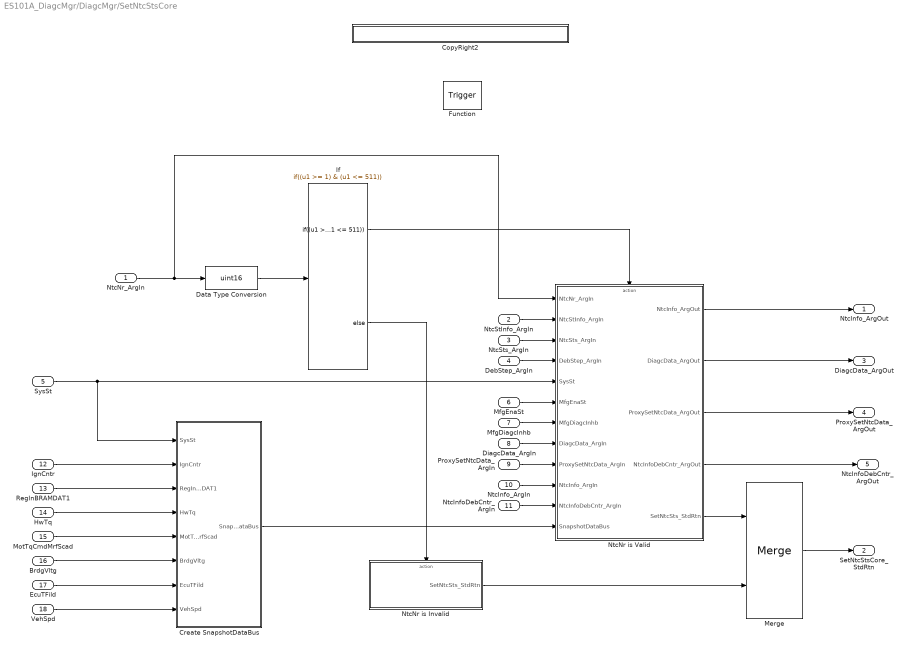
== system ES101A_DiagcMgr/DiagcMgr/SetNtcStsCore ==
  NtcNr_ArgIn : Inport  OutDataTypeStr=Enum: NtcNr1
  NtcStInfo_ArgIn : Inport  Port=2
  NtcSts_ArgIn : Inport  Port=3
  DebStep_ArgIn : Inport  Port=4
  SysSt : Inport  Port=5
  MfgEnaSt : Inport  Port=6
  MfgDiagcInhb : Inport  Port=7
  DiagcData_ArgIn : Inport  Port=8
  ProxySetNtcData_ArgIn : Inport  Port=9
  NtcInfo_ArgIn : Inport  Port=10
  NtcInfoDebCntr_ArgIn : Inport  Port=11
  IgnCntr : Inport  Port=12
  RegInBRAMDAT1 : Inport  Port=13
  HwTq : Inport  Port=14
  MotTqCmdMrfScad : Inport  Port=15
  BrdgVltg : Inport  Port=16
  EcuTFild : Inport  Port=17
  VehSpd : Inport  Port=18
  Function : TriggerPort  TriggerType=function-call  OutputDataType=double
  CopyRight2 : Subsystem  Description=|  mask(Copyright Information){none=on}
      | Copyright info block.                                               
      |                                                                     
      | Place copyright information at the top of every subsystem in design.
      mask prompts: none "No parameters"
      mask help: Place copyright information at the top of every subsystem in design.
      mask Display:
      | NxtrConf = 'Nexteer Confidential';
      | 
      | sys = bdroot; %handle for the current model ("system")
      | first = get_param(sys,'Created');
      | first = first(end-3:end);  %year is last four digits
      | 
      | last = get_param(sys,'LastModifiedDate');
      | if isempty(last)
      |     last = datestr(now,'yyyy');
      | else
      |     last = last(end-3:end);
      | end
      | 
      | if strcmp(first,last)
      |     fprintf('%s -- Copyright %s Nexteer',NxtrConf,first)
      | else
      |     fprintf('%s -- %s%s- %s Nexteer',NxtrConf,char(169),first,last)
      | end
  Create SnapshotDataBus : Subsystem  RequirementInfo="{'linktype_rmi_doors' '0000c474 (/ESG Group/FDD Module Requirements/EA4 Specific/ES101A_DiagcMgr)' '#ES101A_341' 'true' 'REQ:  ES101A_341' '' } %GIDa_ba4124e0_3fab_4f8e_9fd9_197771b46e65"
  Data Type Conversion : DataTypeConversion  OutDataTypeStr=uint16
  If : If  IfExpression=(u1 >= 1) & (u1 <= 511)
  Merge : Merge
  NtcNr is Invalid : Subsystem  TreatAsAtomicUnit=on
  NtcNr is Valid : Subsystem  RequirementInfo="{'linktype_rmi_doors' '0000c474 (/ESG Group/FDD Module Requirements/EA4 Specific/ES101A_DiagcMgr)' '#ES101A_278' 'true' 'REQ:  ES101A_278' '' ; 'linktype_rmi_doors' '0000c474 (/ESG Group/FDD Module Requirements/EA4 Specific/ES101A_DiagcMgr)' '#ES101A_279' 'true' 'REQ:  ES101A_279' '' } %GIDa_60efcd41_1012_4355_bd94_61ad27d99b58"
  "NtcInfo_ArgOut " : Outport
  SetNtcStsCore_StdRtn : Outport  Port=2
  "DiagcData_ArgOut " : Outport  Port=3
  "ProxySetNtcData_ArgOut " : Outport  Port=4
  "NtcInfoDebCntr_ArgOut " : Outport  Port=5
  wires:
  If/1 -> NtcNr is Valid/Action
  If/2 -> NtcNr is Invalid/Action
  NtcNr_ArgIn/1 -> NtcNr is Valid/1(NtcNr_ArgIn), Data Type Conversion/1
  NtcStInfo_ArgIn/1 -> NtcNr is Valid/2(NtcStInfo_ArgIn)
  NtcSts_ArgIn/1 -> NtcNr is Valid/3(NtcSts_ArgIn)
  DebStep_ArgIn/1 -> NtcNr is Valid/4(DebStep_ArgIn)
  Data Type Conversion/1 -> If/1
  SysSt/1 -> Create SnapshotDataBus/1(SysSt), NtcNr is Valid/5(SysSt)
  MfgDiagcInhb/1 -> NtcNr is Valid/7(MfgDiagcInhb)
  DiagcData_ArgIn/1 -> NtcNr is Valid/8(DiagcData_ArgIn)
  ProxySetNtcData_ArgIn/1 -> NtcNr is Valid/9(ProxySetNtcData_ArgIn)
  NtcInfo_ArgIn/1 -> NtcNr is Valid/10(NtcInfo_ArgIn)
  NtcNr is Valid/1(NtcInfo_ArgOut) -> "NtcInfo_ArgOut "/1
  Merge/1 -> SetNtcStsCore_StdRtn/1
  NtcNr is Valid/5(SetNtcSts_StdRtn) -> Merge/1
  NtcNr is Invalid/1(SetNtcSts_StdRtn) -> Merge/2
  NtcNr is Valid/2(DiagcData_ArgOut) -> "DiagcData_ArgOut "/1
  NtcNr is Valid/3(ProxySetNtcData_ArgOut) -> "ProxySetNtcData_ArgOut "/1
  NtcInfoDebCntr_ArgIn/1 -> NtcNr is Valid/11(NtcInfoDebCntr_ArgIn)
  NtcNr is Valid/4(NtcInfoDebCntr_ArgOut) -> "NtcInfoDebCntr_ArgOut "/1
  MfgEnaSt/1 -> NtcNr is Valid/6(MfgEnaSt)
  IgnCntr/1 -> Create SnapshotDataBus/2(IgnCntr)
  RegInBRAMDAT1/1 -> Create SnapshotDataBus/3(RegInBRAMDAT1)
  HwTq/1 -> Create SnapshotDataBus/4(HwTq)
  MotTqCmdMrfScad/1 -> Create SnapshotDataBus/5(MotTqCmdMrfScad)
  BrdgVltg/1 -> Create SnapshotDataBus/6(BrdgVltg)
  EcuTFild/1 -> Create SnapshotDataBus/7(EcuTFild)
  VehSpd/1 -> Create SnapshotDataBus/8(VehSpd)
  Create SnapshotDataBus/1(SnapshotDataBus) -> NtcNr is Valid/12(SnapshotDataBus)

== system ES101A_DiagcMgr/DiagcMgr/UpdDtcEnaCdn ==
  DtcEnaCdnSts_ArgIn : Inport
  DtcEnaCdnId_ArgIn : Inport  Port=2
  Function : TriggerPort  TriggerType=function-call
  ClrBit : Subsystem  TreatAsAtomicUnit=on
  CopyRight2 : Subsystem  Description=|  mask(Copyright Information){none=on}
      | Copyright info block.                                               
      |                                                                     
      | Place copyright information at the top of every subsystem in design.
      mask prompts: none "No parameters"
      mask help: Place copyright information at the top of every subsystem in design.
      mask Display:
      | NxtrConf = 'Nexteer Confidential';
      | 
      | sys = bdroot; %handle for the current model ("system")
      | first = get_param(sys,'Created');
      | first = first(end-3:end);  %year is last four digits
      | 
      | last = get_param(sys,'LastModifiedDate');
      | if isempty(last)
      |     last = datestr(now,'yyyy');
      | else
      |     last = last(end-3:end);
      | end
      | 
      | if strcmp(first,last)
      |     fprintf('%s -- Copyright %s Nexteer',NxtrConf,first)
      | else
      |     fprintf('%s -- %s%s- %s Nexteer',NxtrConf,char(169),first,last)
      | end
  If : If  IfExpression=u1 == 1
  SetBit : Subsystem  TreatAsAtomicUnit=on
  wires:
  DtcEnaCdnSts_ArgIn/1 -> If/1
  If/1 -> SetBit/Action
  If/2 -> ClrBit/Action
  DtcEnaCdnId_ArgIn/1 -> ClrBit/1(DtcEnaCdnId_ArgIn), SetBit/1(DtcEnaCdnId_ArgIn)

== system ES101A_DiagcMgr/DiagcMgr/ClrAllDiagc/CopyRight2 ==

== system ES101A_DiagcMgr/DiagcMgr/ClrAllDiagc/If Action Subsystem ==
  Action Port : ActionPort  ActionType=then
  Clear : Constant  Value=0
  ClrDiagcFlg : Outport
  wires:
  Clear/1 -> ClrDiagcFlg/1
